simulink model "simulink"  (R2024a)
settings: Solver=VariableStepAuto  StartTime=0.0  StopTime=10.0  RelTol=1e-3
settings Model: Creator=victus  LastModifiedBy=victus

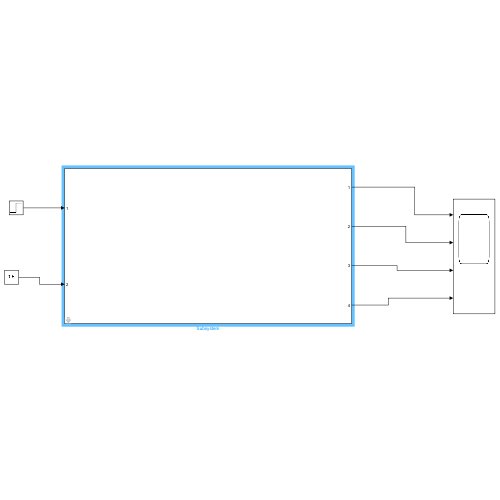
[thumbnail: Simulink's stored preview of the top-level diagram]
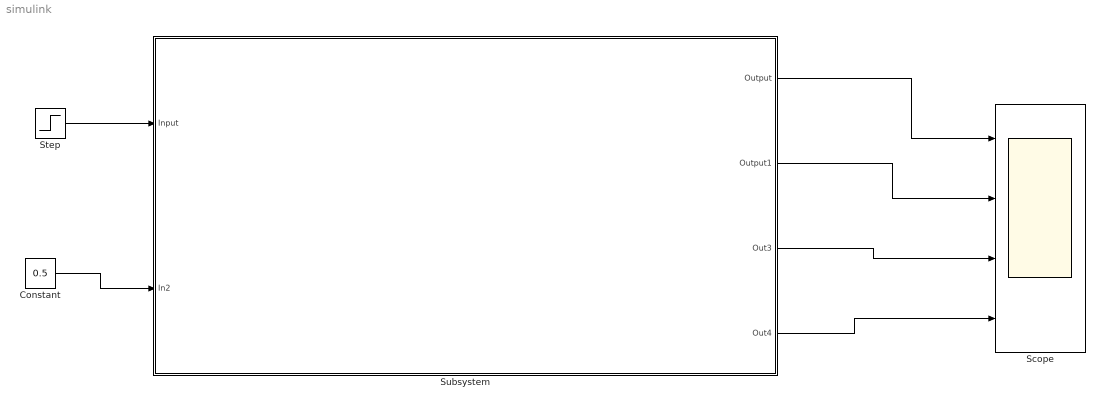
== system simulink ==
  Constant : Constant  Value=0.5
  Scope : Scope  NumInputPorts=4
  Step : Step  After=5  SampleTime=0
  Subsystem : Subsystem  mask{Js=0.5, Jm=0.1, Bm=0.01, Bs=0.2, Im=20, Ks=50}
  wires:
  Subsystem/3(Out3) -> Scope/3
  Subsystem/4(Out4) -> Scope/4
  Step/1 -> Subsystem/1(Input)
  Constant/1 -> Subsystem/2(In2)
  Subsystem/2(Output1) -> Scope/2
  Subsystem/1(Output) -> Scope/1

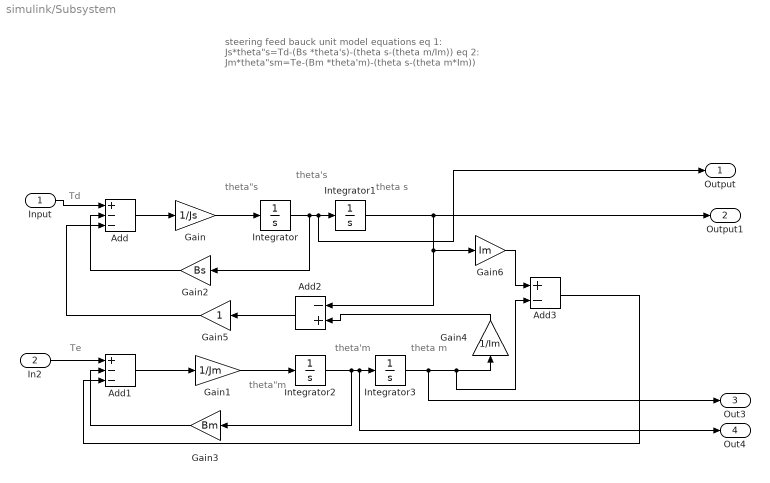
== system simulink/Subsystem ==
  note: steering feed bauck unit model equations
      | eq 1:
      | Js*theta"s=Td-(Bs *theta's)-(theta s-(theta m/Im))
      | eq 2:
      | Jm*theta"sm=Te-(Bm *theta'm)-(theta s-(theta m*Im))
  note: theta"s
  note: theta m
  note: theta"m
  note: Te
  note: theta s
  note: theta's
  note: Td
  note: theta'm
  Input : Inport
  In2 : Inport  Port=2
  Add : Sum  Inputs=+--
  Add1 : Sum  Inputs=+--
  Add2 : Sum  Inputs=-+
  Add3 : Sum  Inputs=+-
  Gain : Gain  Gain=1/Js
  Gain1 : Gain  Gain=1/Jm
  Gain2 : Gain  Gain=Bs
  Gain3 : Gain  Gain=Bm
  Gain4 : Gain  Gain=1/Im
  Gain5 : Gain
  Gain6 : Gain  Gain=Im
  Integrator{,1..3} (4 alike) : Integrator
  Output : Outport
  Output1 : Outport  Port=2
  Out3 : Outport  Port=3
  Out4 : Outport  Port=4
  wires:
  Integrator/1 -> Gain2/1, Output/1, Integrator1/1
  Integrator1/1 -> Output1/1, Add2/1, Gain6/1
  Integrator2/1 -> Gain3/1, Out4/1, Integrator3/1
  Gain4/1 -> Add2/2
  Integrator3/1 -> Out3/1, Gain4/1, Add3/2
  Gain/1 -> Integrator/1
  Add/1 -> Gain/1
  Gain2/1 -> Add/2
  Gain5/1 -> Add/3
  Add3/1 -> Add1/3
  Gain6/1 -> Add3/1
  Gain1/1 -> Integrator2/1
  Add1/1 -> Gain1/1
  Add2/1 -> Gain5/1
  Gain3/1 -> Add1/2
  In2/1 -> Add1/1
  Input/1 -> Add/1
